simulink model "thruster_model"  (R2020a)
settings: Solver=FixedStepAuto  StartTime=0.0  StopTime=10.0  FixedStep=0.01  RelTol=1e-3
PreLoadFcn:
  | load("interfaces.mat");
libraries: simulink_extras x8, simulink x4
settings Model: Creator=thomas.evang  LastModifiedBy=thomas.evang
settings SFSimCC: CustomCodeUndefinedFunction=UseInterfaceOnly
settings RTWCC: Description=Generic Real-Time Target  RetainRTWFile=on

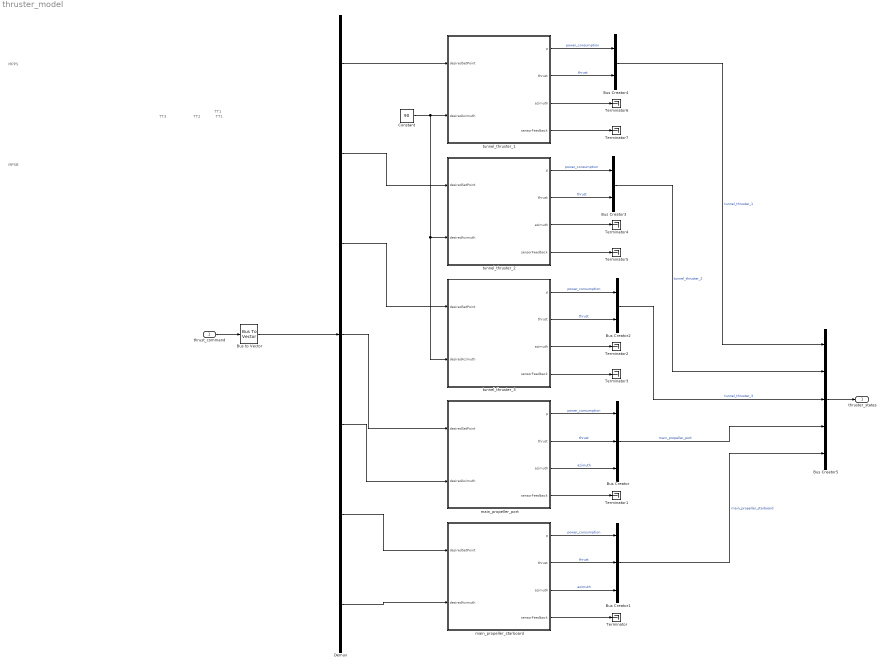
== system thruster_model ==
  note: TT1
  note: TT3
  note: TT1
  note: MPPS
  note: TT2
  note: MPSB
  thrust_command : Inport  OutDataTypeStr=Bus: thrust_command
  Bus Creator : BusCreator  Inputs=3
  Bus Creator1 : BusCreator  Inputs=3
  Bus Creator2 : BusCreator  Inputs=2
  Bus Creator3 : BusCreator  Inputs=2
  Bus Creator4 : BusCreator  Inputs=2
  Bus Creator5 : BusCreator  Inputs=5  OutDataTypeStr=Bus: thruster_states
  Bus to Vector : BusToVector
  Constant : Constant  Value=90
  Demux : Demux  Outputs=7
  Terminator{,1..7} (8 alike) : Terminator
  main_propeller_port : Subsystem
  main_propeller_starboard : Subsystem
  tunnel_thruster_1 : Subsystem
  tunnel_thruster_2 : Subsystem
  tunnel_thruster_3 : Subsystem
  thruster_states : Outport  OutDataTypeStr=Bus: thruster_states  VectorParamsAs1DForOutWhenUnconnected=off
  wires:
  Bus Creator1/1 -> Bus Creator5/5  "main_propeller_starboard"
  Bus Creator2/1 -> Bus Creator5/3  "tunnel_thruster_3"
  Demux/1 -> tunnel_thruster_1/1(desiredSetPoint)
  tunnel_thruster_1/4(sensorFeedback) -> Terminator7/1
  thrust_command/1 -> Bus to Vector/1
  tunnel_thruster_3/4(sensorFeedback) -> Terminator3/1
  Demux/3 -> tunnel_thruster_3/1(desiredSetPoint)
  main_propeller_starboard/4(sensorFeedback) -> Terminator/1
  Constant/1 -> tunnel_thruster_3/2(desiredAzimuth), tunnel_thruster_2/2(desiredAzimuth), tunnel_thruster_1/2(desiredAzimuth)
  main_propeller_port/4(sensorFeedback) -> Terminator1/1
  tunnel_thruster_1/3(azimuth) -> Terminator6/1
  main_propeller_starboard/2(thrust) -> Bus Creator1/2  "thrust"
  tunnel_thruster_3/3(azimuth) -> Terminator2/1
  tunnel_thruster_3/1(p) -> Bus Creator2/1  "power_consumption"
  Demux/4 -> main_propeller_port/1(desiredSetPoint)
  main_propeller_port/2(thrust) -> Bus Creator/2  "thrust"
  Demux/2 -> tunnel_thruster_2/1(desiredSetPoint)
  tunnel_thruster_2/4(sensorFeedback) -> Terminator5/1
  Bus Creator5/1 -> thruster_states/1
  tunnel_thruster_3/2(thrust) -> Bus Creator2/2  "thrust"
  Demux/5 -> main_propeller_port/2(desiredAzimuth)
  Bus Creator3/1 -> Bus Creator5/2  "tunnel_thruster_2"
  Bus Creator4/1 -> Bus Creator5/1  "tunnel_thruster_1"
  Demux/6 -> main_propeller_starboard/1(desiredSetPoint)
  Bus Creator/1 -> Bus Creator5/4  "main_propeller_port"
  main_propeller_starboard/1(p) -> Bus Creator1/1  "power_consumption"
  main_propeller_starboard/3(azimuth) -> Bus Creator1/3  "azimuth"
  main_propeller_port/1(p) -> Bus Creator/1  "power_consumption"
  tunnel_thruster_1/2(thrust) -> Bus Creator4/2  "thrust"
  tunnel_thruster_2/1(p) -> Bus Creator3/1  "power_consumption"
  tunnel_thruster_2/2(thrust) -> Bus Creator3/2  "thrust"
  tunnel_thruster_1/1(p) -> Bus Creator4/1  "power_consumption"
  Demux/7 -> main_propeller_starboard/2(desiredAzimuth)
  main_propeller_port/3(azimuth) -> Bus Creator/3  "azimuth"
  tunnel_thruster_2/3(azimuth) -> Terminator4/1
  Bus to Vector/1 -> Demux/1

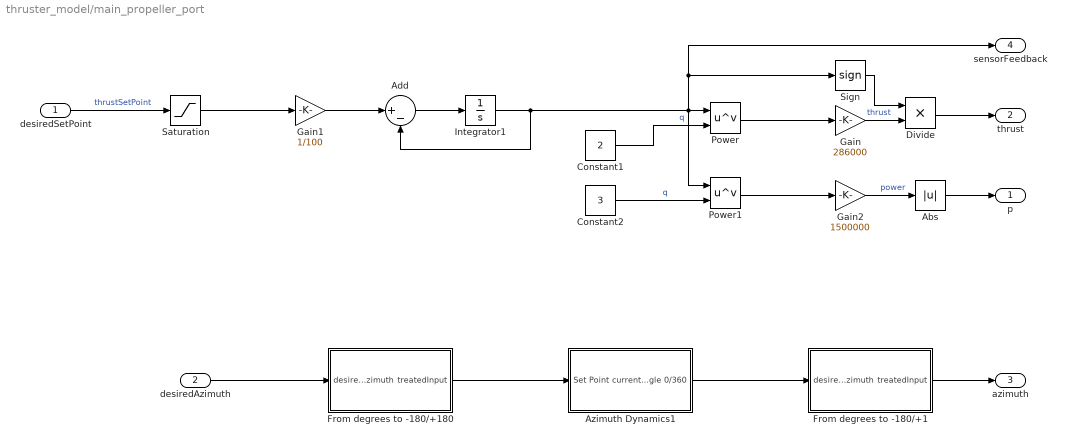
== system thruster_model/main_propeller_port ==
  desiredSetPoint : Inport  Unit=N
  desiredAzimuth : Inport  Port=2  Unit=deg
  Abs : Abs
  Add : Sum  Inputs=|+-
  Azimuth Dynamics1 : Subsystem
  Constant1 : Constant  Value=2
  Constant2 : Constant  Value=3
  Divide : Product
  From degrees to -180/+1 : Subsystem
  From degrees to -180/+180 : Subsystem
  Gain : Gain  Gain=286000
  Gain1 : Gain  Gain=1/100
  Gain2 : Gain  Gain=1500000
  Integrator1 : Integrator
  Power : Math  Operator=pow  SignedPower=on  SaturateOnIntegerOverflow=on
  Power1 : Math  Operator=pow  SignedPower=on  SaturateOnIntegerOverflow=on
  Saturation : Saturate  UpperLimit=100  LowerLimit=-100
  Sign : Signum
  p : Outport  Unit=W  VectorParamsAs1DForOutWhenUnconnected=off  BusOutputAsStruct=on
  thrust : Outport  Port=2  Unit=N  VectorParamsAs1DForOutWhenUnconnected=off
  azimuth : Outport  Port=3  Unit=deg  VectorParamsAs1DForOutWhenUnconnected=off  BusOutputAsStruct=on
  sensorFeedback : Outport  Port=4  Unit=deg  VectorParamsAs1DForOutWhenUnconnected=off  BusOutputAsStruct=on
  wires:
  Gain1/1 -> Add/1
  From degrees to -180/+180/1(treatedInput) -> Azimuth Dynamics1/1(Set Point)
  Add/1 -> Integrator1/1
  Saturation/1 -> Gain1/1
  Divide/1 -> thrust/1
  Power1/1 -> Gain2/1
  desiredSetPoint/1 -> Saturation/1  "thrustSetPoint"
  Power/1 -> Gain/1
  Azimuth Dynamics1/1(currentAngle 0/360) -> From degrees to -180/+1/1(desiredAzimuth)
  Gain/1 -> Divide/2  "thrust"
  From degrees to -180/+1/1(treatedInput) -> azimuth/1
  Gain2/1 -> Abs/1  "power"
  Constant2/1 -> Power1/2  "q"
  Sign/1 -> Divide/1
  Constant1/1 -> Power/2  "q"
  Abs/1 -> p/1
  desiredAzimuth/1 -> From degrees to -180/+180/1(desiredAzimuth)
  Integrator1/1 -> Power/1, Power1/1, sensorFeedback/1, Sign/1, Add/2

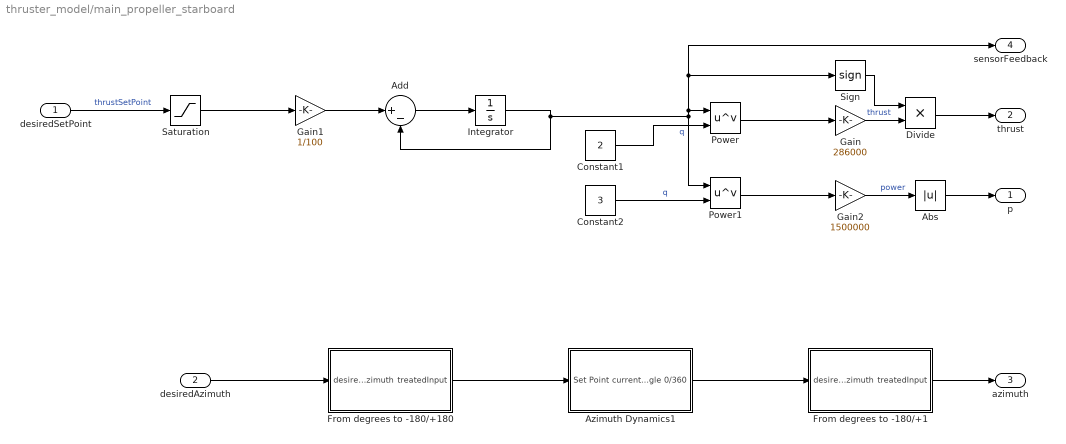
== system thruster_model/main_propeller_starboard ==
  desiredSetPoint : Inport  Unit=N
  desiredAzimuth : Inport  Port=2  Unit=deg
  Abs : Abs
  Add : Sum  Inputs=|+-
  Azimuth Dynamics1 : Subsystem
  Constant1 : Constant  Value=2
  Constant2 : Constant  Value=3
  Divide : Product
  From degrees to -180/+1 : Subsystem
  From degrees to -180/+180 : Subsystem
  Gain : Gain  Gain=286000
  Gain1 : Gain  Gain=1/100
  Gain2 : Gain  Gain=1500000
  Integrator : Integrator
  Power : Math  Operator=pow  SignedPower=on  SaturateOnIntegerOverflow=on
  Power1 : Math  Operator=pow  SignedPower=on  SaturateOnIntegerOverflow=on
  Saturation : Saturate  UpperLimit=100  LowerLimit=-100
  Sign : Signum
  p : Outport  Unit=W  VectorParamsAs1DForOutWhenUnconnected=off  BusOutputAsStruct=on
  thrust : Outport  Port=2  Unit=N  VectorParamsAs1DForOutWhenUnconnected=off
  azimuth : Outport  Port=3  Unit=deg  VectorParamsAs1DForOutWhenUnconnected=off  BusOutputAsStruct=on
  sensorFeedback : Outport  Port=4  Unit=deg  VectorParamsAs1DForOutWhenUnconnected=off  BusOutputAsStruct=on
  wires:
  desiredAzimuth/1 -> From degrees to -180/+180/1(desiredAzimuth)
  Abs/1 -> p/1
  Constant1/1 -> Power/2  "q"
  Sign/1 -> Divide/1
  Constant2/1 -> Power1/2  "q"
  Gain2/1 -> Abs/1  "power"
  From degrees to -180/+1/1(treatedInput) -> azimuth/1
  Gain/1 -> Divide/2  "thrust"
  Azimuth Dynamics1/1(currentAngle 0/360) -> From degrees to -180/+1/1(desiredAzimuth)
  Power/1 -> Gain/1
  desiredSetPoint/1 -> Saturation/1  "thrustSetPoint"
  Power1/1 -> Gain2/1
  Divide/1 -> thrust/1
  Saturation/1 -> Gain1/1
  Add/1 -> Integrator/1
  From degrees to -180/+180/1(treatedInput) -> Azimuth Dynamics1/1(Set Point)
  Gain1/1 -> Add/1
  Integrator/1 -> Sign/1, sensorFeedback/1, Power/1, Power1/1, Add/2

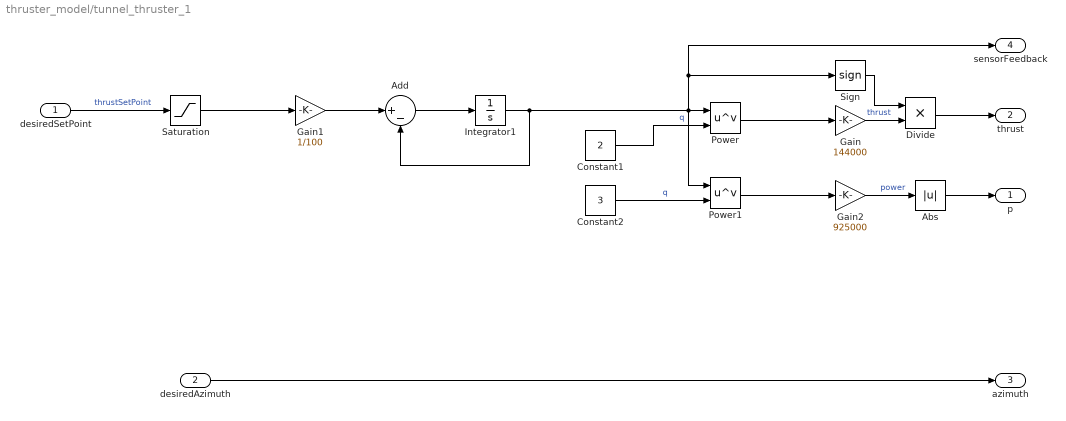
== system thruster_model/tunnel_thruster_1 ==
  desiredSetPoint : Inport  Unit=N
  desiredAzimuth : Inport  Port=2  Unit=deg
  Abs : Abs
  Add : Sum  Inputs=|+-
  Constant1 : Constant  Value=2
  Constant2 : Constant  Value=3
  Divide : Product
  Gain : Gain  Gain=144000
  Gain1 : Gain  Gain=1/100
  Gain2 : Gain  Gain=925000
  Integrator1 : Integrator
  Power : Math  Operator=pow  SignedPower=on  SaturateOnIntegerOverflow=on
  Power1 : Math  Operator=pow  SignedPower=on  SaturateOnIntegerOverflow=on
  Saturation : Saturate  UpperLimit=100  LowerLimit=-100
  Sign : Signum
  p : Outport  Unit=W  VectorParamsAs1DForOutWhenUnconnected=off  BusOutputAsStruct=on
  thrust : Outport  Port=2  Unit=N  VectorParamsAs1DForOutWhenUnconnected=off
  azimuth : Outport  Port=3  Unit=deg  VectorParamsAs1DForOutWhenUnconnected=off  BusOutputAsStruct=on
  sensorFeedback : Outport  Port=4  Unit=deg  VectorParamsAs1DForOutWhenUnconnected=off  BusOutputAsStruct=on
  wires:
  Abs/1 -> p/1
  Constant1/1 -> Power/2  "q"
  Sign/1 -> Divide/1
  Constant2/1 -> Power1/2  "q"
  Gain2/1 -> Abs/1  "power"
  Gain/1 -> Divide/2  "thrust"
  Power/1 -> Gain/1
  desiredSetPoint/1 -> Saturation/1  "thrustSetPoint"
  Power1/1 -> Gain2/1
  Divide/1 -> thrust/1
  Saturation/1 -> Gain1/1
  Integrator1/1 -> Add/2, Sign/1, sensorFeedback/1, Power1/1, Power/1
  Add/1 -> Integrator1/1
  Gain1/1 -> Add/1
  desiredAzimuth/1 -> azimuth/1

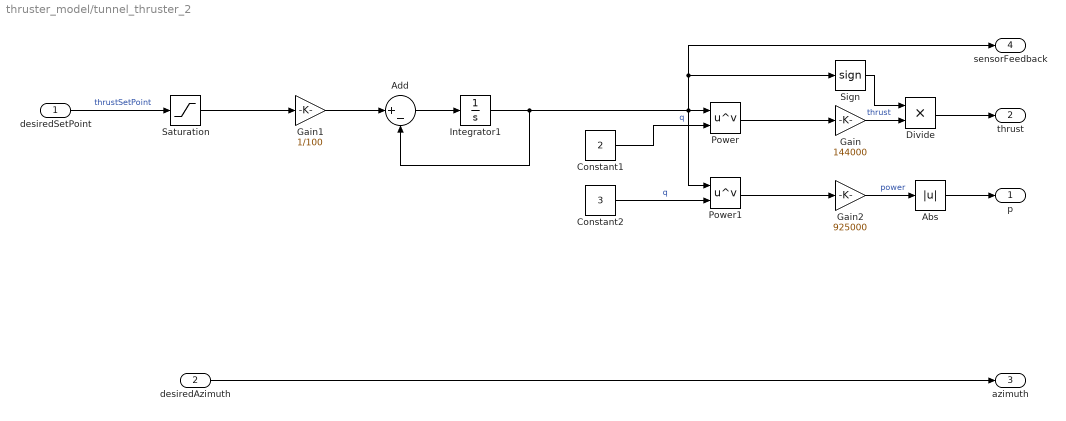
== system thruster_model/tunnel_thruster_2 ==
  desiredSetPoint : Inport  Unit=N
  desiredAzimuth : Inport  Port=2  Unit=deg
  Abs : Abs
  Add : Sum  Inputs=|+-
  Constant1 : Constant  Value=2
  Constant2 : Constant  Value=3
  Divide : Product
  Gain : Gain  Gain=144000
  Gain1 : Gain  Gain=1/100
  Gain2 : Gain  Gain=925000
  Integrator1 : Integrator
  Power : Math  Operator=pow  SignedPower=on  SaturateOnIntegerOverflow=on
  Power1 : Math  Operator=pow  SignedPower=on  SaturateOnIntegerOverflow=on
  Saturation : Saturate  UpperLimit=100  LowerLimit=-100
  Sign : Signum
  p : Outport  Unit=W  VectorParamsAs1DForOutWhenUnconnected=off  BusOutputAsStruct=on
  thrust : Outport  Port=2  Unit=N  VectorParamsAs1DForOutWhenUnconnected=off
  azimuth : Outport  Port=3  Unit=deg  VectorParamsAs1DForOutWhenUnconnected=off  BusOutputAsStruct=on
  sensorFeedback : Outport  Port=4  Unit=deg  VectorParamsAs1DForOutWhenUnconnected=off  BusOutputAsStruct=on
  wires:
  Gain1/1 -> Add/1
  Add/1 -> Integrator1/1
  Integrator1/1 -> Add/2, Power/1, Power1/1, sensorFeedback/1, Sign/1
  Saturation/1 -> Gain1/1
  Divide/1 -> thrust/1
  Power1/1 -> Gain2/1
  desiredSetPoint/1 -> Saturation/1  "thrustSetPoint"
  Power/1 -> Gain/1
  Gain/1 -> Divide/2  "thrust"
  Gain2/1 -> Abs/1  "power"
  Constant2/1 -> Power1/2  "q"
  Sign/1 -> Divide/1
  Constant1/1 -> Power/2  "q"
  Abs/1 -> p/1
  desiredAzimuth/1 -> azimuth/1

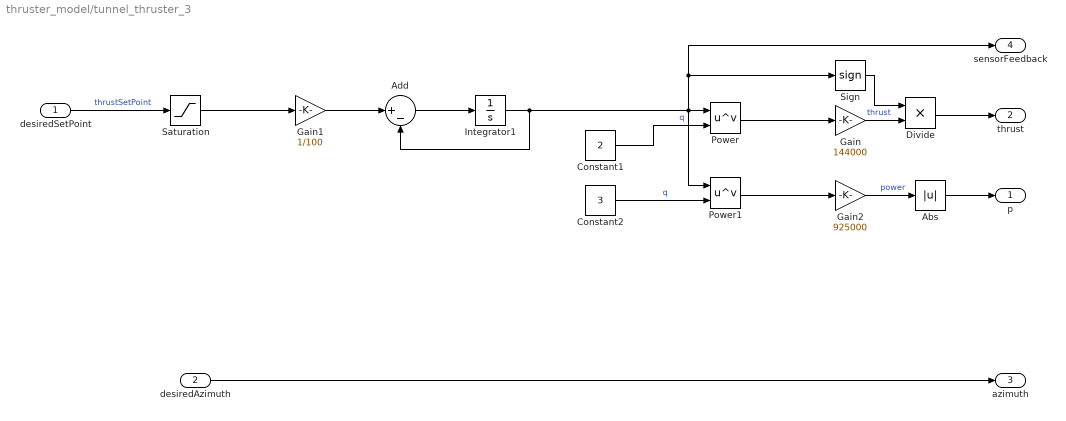
== system thruster_model/tunnel_thruster_3 ==
  desiredSetPoint : Inport  Unit=N
  desiredAzimuth : Inport  Port=2  Unit=deg
  Abs : Abs
  Add : Sum  Inputs=|+-
  Constant1 : Constant  Value=2
  Constant2 : Constant  Value=3
  Divide : Product
  Gain : Gain  Gain=144000
  Gain1 : Gain  Gain=1/100
  Gain2 : Gain  Gain=925000
  Integrator1 : Integrator
  Power : Math  Operator=pow  SignedPower=on  SaturateOnIntegerOverflow=on
  Power1 : Math  Operator=pow  SignedPower=on  SaturateOnIntegerOverflow=on
  Saturation : Saturate  UpperLimit=100  LowerLimit=-100
  Sign : Signum
  p : Outport  Unit=W  VectorParamsAs1DForOutWhenUnconnected=off  BusOutputAsStruct=on
  thrust : Outport  Port=2  Unit=N  VectorParamsAs1DForOutWhenUnconnected=off
  azimuth : Outport  Port=3  Unit=deg  VectorParamsAs1DForOutWhenUnconnected=off  BusOutputAsStruct=on
  sensorFeedback : Outport  Port=4  Unit=deg  VectorParamsAs1DForOutWhenUnconnected=off  BusOutputAsStruct=on
  wires:
  Abs/1 -> p/1
  Constant1/1 -> Power/2  "q"
  Sign/1 -> Divide/1
  Constant2/1 -> Power1/2  "q"
  Gain2/1 -> Abs/1  "power"
  Gain/1 -> Divide/2  "thrust"
  Power/1 -> Gain/1
  desiredSetPoint/1 -> Saturation/1  "thrustSetPoint"
  Power1/1 -> Gain2/1
  Divide/1 -> thrust/1
  Saturation/1 -> Gain1/1
  Integrator1/1 -> Add/2, Sign/1, sensorFeedback/1, Power1/1, Power/1
  Add/1 -> Integrator1/1
  Gain1/1 -> Add/1
  desiredAzimuth/1 -> azimuth/1

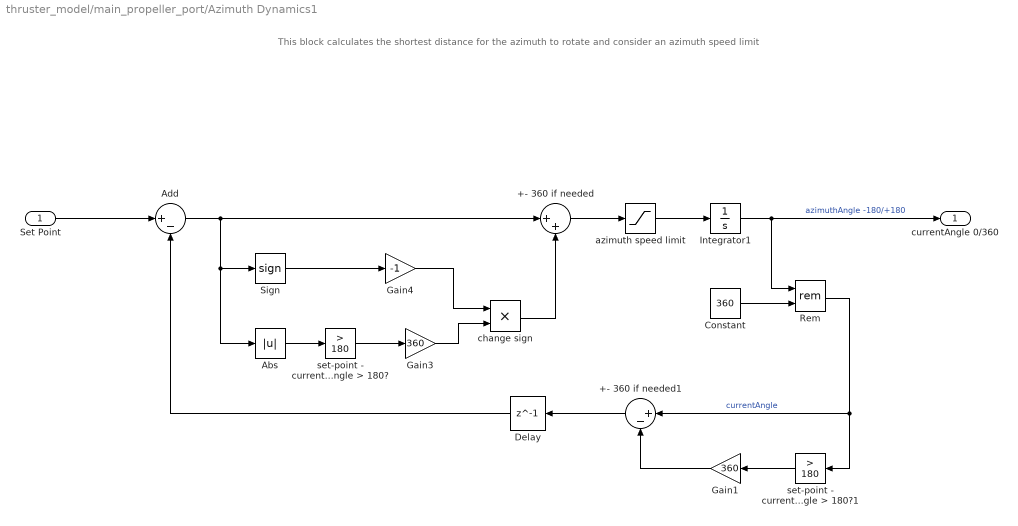
== system thruster_model/main_propeller_port/Azimuth Dynamics1 ==
  note: This block calculates the shortest distance for the azimuth to rotate and consider an azimuth speed limit
  Set Point : Inport
  +- 360 if needed : Sum  Inputs=|++
  +- 360 if needed1 : Sum  Inputs=|+-
  Abs : Abs
  Add : Sum  Inputs=|+-
  Constant : Constant  Value=360
  Delay : Delay  DelayLength=1
  Gain1 : Gain  Gain=360
  Gain3 : Gain  Gain=360
  Gain4 : Gain  Gain=-1
  Integrator1 : Integrator  WrappedStateUpperValue=180  WrappedStateLowerValue=-180
  Rem : Math  Operator=rem  SignedPower=on  SaturateOnIntegerOverflow=on
  Sign : Signum
  azimuth speed limit : Saturate  UpperLimit=180  LowerLimit=-180
  change sign : Product
  set-point - currentAngle > 180? : simulink/Logic and Bit Operations/Compare To Constant  relop=>  const=180  OutDataTypeStr=boolean
  set-point - currentAngle > 180?1 : simulink/Logic and Bit Operations/Compare To Constant  relop=>  const=180  OutDataTypeStr=boolean
  currentAngle 0/360 : Outport  VectorParamsAs1DForOutWhenUnconnected=off
  wires:
  +- 360 if needed1/1 -> Delay/1
  set-point - currentAngle > 180?1/1 -> Gain1/1
  Gain1/1 -> +- 360 if needed1/2
  Abs/1 -> set-point - currentAngle > 180?/1
  Rem/1 -> +- 360 if needed1/1, set-point - currentAngle > 180?1/1  "currentAngle"
  set-point - currentAngle > 180?/1 -> Gain3/1
  Delay/1 -> Add/2
  Constant/1 -> Rem/2
  azimuth speed limit/1 -> Integrator1/1
  change sign/1 -> +- 360 if needed/2
  Gain4/1 -> change sign/1
  Gain3/1 -> change sign/2
  Sign/1 -> Gain4/1
  Integrator1/1 -> Rem/1, currentAngle 0/360/1  "azimuthAngle -180/+180"
  Set Point/1 -> Add/1
  Add/1 -> +- 360 if needed/1, Abs/1, Sign/1
  +- 360 if needed/1 -> azimuth speed limit/1

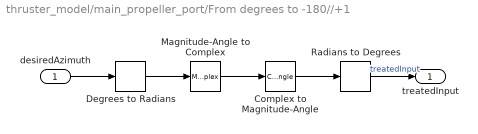
== system thruster_model/main_propeller_port/From degrees to -180//+1 ==
  desiredAzimuth : Inport
  Complex to Magnitude-Angle : ComplexToMagnitudeAngle  Output=Angle
  Degrees to Radians : simulink_extras/Transformations/Degrees to Radians
  Magnitude-Angle to Complex : MagnitudeAngleToComplex  Input=Angle  ConstantPart=1
  Radians to Degrees : simulink_extras/Transformations/Radians to Degrees
  treatedInput : Outport  VectorParamsAs1DForOutWhenUnconnected=off
  wires:
  desiredAzimuth/1 -> Degrees to Radians/1
  Degrees to Radians/1 -> Magnitude-Angle to Complex/1
  Complex to Magnitude-Angle/1 -> Radians to Degrees/1
  Magnitude-Angle to Complex/1 -> Complex to Magnitude-Angle/1
  Radians to Degrees/1 -> treatedInput/1  "treatedInput"

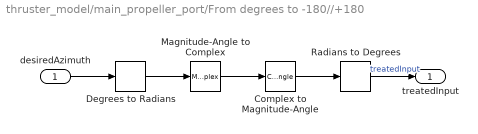
== system thruster_model/main_propeller_port/From degrees to -180//+180 ==
  desiredAzimuth : Inport
  Complex to Magnitude-Angle : ComplexToMagnitudeAngle  Output=Angle
  Degrees to Radians : simulink_extras/Transformations/Degrees to Radians
  Magnitude-Angle to Complex : MagnitudeAngleToComplex  Input=Angle  ConstantPart=1
  Radians to Degrees : simulink_extras/Transformations/Radians to Degrees
  treatedInput : Outport  VectorParamsAs1DForOutWhenUnconnected=off
  wires:
  Radians to Degrees/1 -> treatedInput/1  "treatedInput"
  Magnitude-Angle to Complex/1 -> Complex to Magnitude-Angle/1
  Complex to Magnitude-Angle/1 -> Radians to Degrees/1
  Degrees to Radians/1 -> Magnitude-Angle to Complex/1
  desiredAzimuth/1 -> Degrees to Radians/1

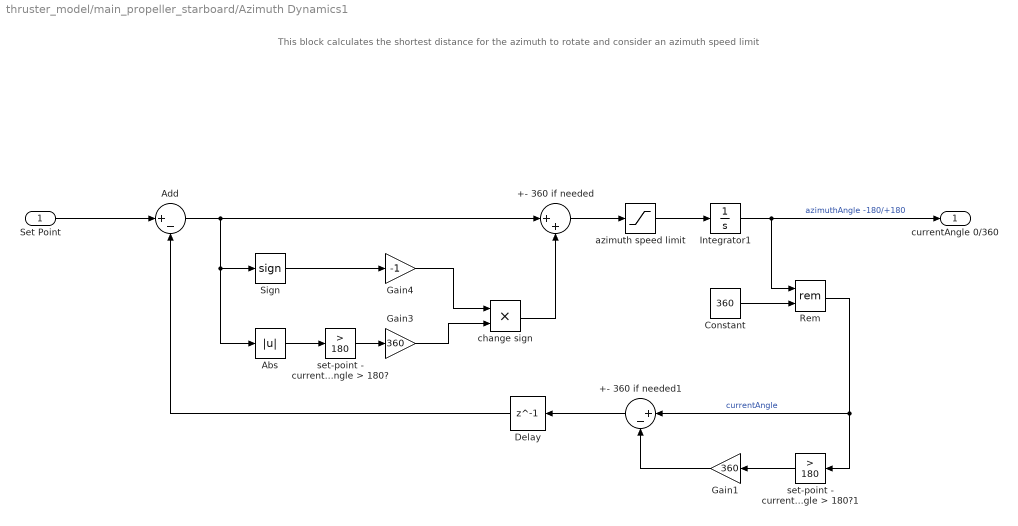
== system thruster_model/main_propeller_starboard/Azimuth Dynamics1 ==
  note: This block calculates the shortest distance for the azimuth to rotate and consider an azimuth speed limit
  Set Point : Inport
  +- 360 if needed : Sum  Inputs=|++
  +- 360 if needed1 : Sum  Inputs=|+-
  Abs : Abs
  Add : Sum  Inputs=|+-
  Constant : Constant  Value=360
  Delay : Delay  DelayLength=1
  Gain1 : Gain  Gain=360
  Gain3 : Gain  Gain=360
  Gain4 : Gain  Gain=-1
  Integrator1 : Integrator  WrappedStateUpperValue=180  WrappedStateLowerValue=-180
  Rem : Math  Operator=rem  SignedPower=on  SaturateOnIntegerOverflow=on
  Sign : Signum
  azimuth speed limit : Saturate  UpperLimit=180  LowerLimit=-180
  change sign : Product
  set-point - currentAngle > 180? : simulink/Logic and Bit Operations/Compare To Constant  relop=>  const=180  OutDataTypeStr=boolean
  set-point - currentAngle > 180?1 : simulink/Logic and Bit Operations/Compare To Constant  relop=>  const=180  OutDataTypeStr=boolean
  currentAngle 0/360 : Outport  VectorParamsAs1DForOutWhenUnconnected=off
  wires:
  +- 360 if needed/1 -> azimuth speed limit/1
  Add/1 -> Sign/1, Abs/1, +- 360 if needed/1
  Set Point/1 -> Add/1
  Integrator1/1 -> currentAngle 0/360/1, Rem/1  "azimuthAngle -180/+180"
  Sign/1 -> Gain4/1
  Gain3/1 -> change sign/2
  Gain4/1 -> change sign/1
  change sign/1 -> +- 360 if needed/2
  azimuth speed limit/1 -> Integrator1/1
  Constant/1 -> Rem/2
  Delay/1 -> Add/2
  set-point - currentAngle > 180?/1 -> Gain3/1
  Rem/1 -> set-point - currentAngle > 180?1/1, +- 360 if needed1/1  "currentAngle"
  Abs/1 -> set-point - currentAngle > 180?/1
  Gain1/1 -> +- 360 if needed1/2
  set-point - currentAngle > 180?1/1 -> Gain1/1
  +- 360 if needed1/1 -> Delay/1

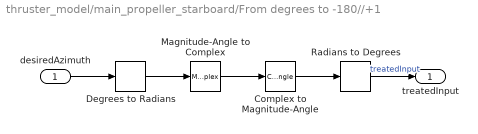
== system thruster_model/main_propeller_starboard/From degrees to -180//+1 ==
  desiredAzimuth : Inport
  Complex to Magnitude-Angle : ComplexToMagnitudeAngle  Output=Angle
  Degrees to Radians : simulink_extras/Transformations/Degrees to Radians
  Magnitude-Angle to Complex : MagnitudeAngleToComplex  Input=Angle  ConstantPart=1
  Radians to Degrees : simulink_extras/Transformations/Radians to Degrees
  treatedInput : Outport  VectorParamsAs1DForOutWhenUnconnected=off
  wires:
  Radians to Degrees/1 -> treatedInput/1  "treatedInput"
  Magnitude-Angle to Complex/1 -> Complex to Magnitude-Angle/1
  Complex to Magnitude-Angle/1 -> Radians to Degrees/1
  Degrees to Radians/1 -> Magnitude-Angle to Complex/1
  desiredAzimuth/1 -> Degrees to Radians/1

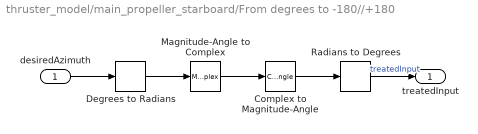
== system thruster_model/main_propeller_starboard/From degrees to -180//+180 ==
  desiredAzimuth : Inport
  Complex to Magnitude-Angle : ComplexToMagnitudeAngle  Output=Angle
  Degrees to Radians : simulink_extras/Transformations/Degrees to Radians
  Magnitude-Angle to Complex : MagnitudeAngleToComplex  Input=Angle  ConstantPart=1
  Radians to Degrees : simulink_extras/Transformations/Radians to Degrees
  treatedInput : Outport  VectorParamsAs1DForOutWhenUnconnected=off
  wires:
  desiredAzimuth/1 -> Degrees to Radians/1
  Degrees to Radians/1 -> Magnitude-Angle to Complex/1
  Complex to Magnitude-Angle/1 -> Radians to Degrees/1
  Magnitude-Angle to Complex/1 -> Complex to Magnitude-Angle/1
  Radians to Degrees/1 -> treatedInput/1  "treatedInput"
